simulink model "two_rotational_mass_flex_shaft_TF"  (R2013b)
settings: Solver=ode45  StartTime=0.0  StopTime=10.0  RelTol=1e-3
values from neighbouring files (symbols this model uses):
  Cw = 1    [two_rotational_mass_flex_coupling.m]
  Jl = 1    [two_rotational_mass_flex_coupling.m]
  Jm = 0.1    [two_rotational_mass_flex_coupling.m]
  Ks = 5    [two_rotational_mass_flex_coupling.m]
settings Model: Creator=User  LastModifiedBy=User

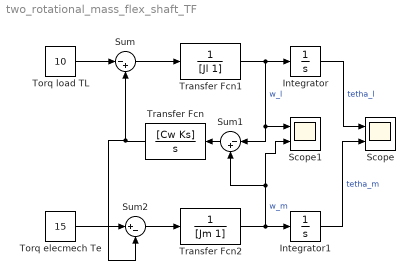
== system two_rotational_mass_flex_shaft_TF ==
  Integrator : Integrator
  Integrator1 : Integrator
  Scope : Scope  NumInputPorts=2
      settings: YMin=-5~-5  YMax=5~5
  Scope1 : Scope  NumInputPorts=2
      settings: YMin=-5~-5  YMax=5~5
  Sum : Sum  Inputs=|-+
  Sum1 : Sum  Inputs=|-+
  Sum2 : Sum  Inputs=|+-
  Torq elecmech Te : Constant  Value=15
  Torq load TL : Constant  Value=10
  Transfer Fcn : TransferFcn  Numerator=[Cw Ks]  Denominator=[1 0]
  Transfer Fcn1 : TransferFcn  Denominator=[Jl 1]
  Transfer Fcn2 : TransferFcn  Denominator=[Jm 1]
  wires:
  Torq load TL/1 -> Sum/1
  Sum/1 -> Transfer Fcn1/1
  Transfer Fcn1/1 -> Scope1/1, Sum1/1, Integrator/1  "w_l"
  Sum1/1 -> Transfer Fcn/1
  Transfer Fcn2/1 -> Integrator1/1, Scope1/2, Sum1/2  "w_m"
  Torq elecmech Te/1 -> Sum2/1
  Sum2/1 -> Transfer Fcn2/1
  Integrator/1 -> Scope/1  "tetha_l"
  Integrator1/1 -> Scope/2  "tetha_m"
  Transfer Fcn/1 -> Sum2/2, Sum/2
